simulink model "test_lcl"  (R2021a)
settings: Solver=VariableStepAuto  StartTime=0.0  StopTime=0.2  RelTol=1e-3
values from neighbouring files (symbols this model uses):
  C_a = 1e-3    (= 0.001)    [init.m]
  Lc_a = 0.1    [init.m]
  Lg_a = 1    [init.m]
  Rc_a = 1    [init.m]
  Rf_a = 0.1    [init.m]
  Rg_a = 1    [init.m]
libraries: spsThreePhaseSeriesRLCBranchLib x4, spsThreePhaseVIMeasurementLib x3, spsThreePhaseSourceLib x2, spsMultimeterLib x1, spspowerguiLib x1
settings Model: Creator=viliv  LastModifiedBy=viliv

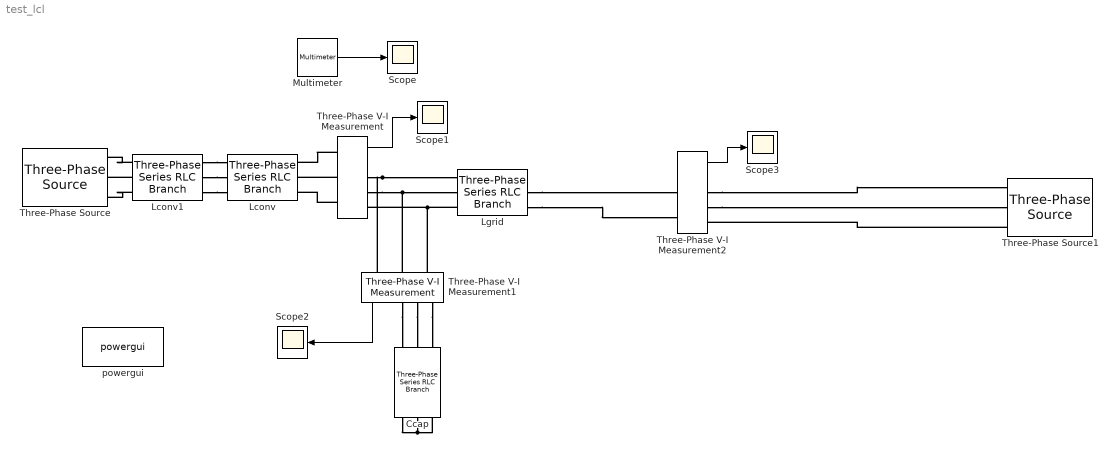
== system test_lcl ==
  Ccap : spsThreePhaseSeriesRLCBranchLib/Three-Phase Series RLC Branch  LConnTagsString=A|B|C  RConnTagsString=A|B|C  BranchType=RC  Resistance=Rf_a  Inductance=2  Capacitance=C_a  Measurements=Branch voltages and currents
  Lconv : spsThreePhaseSeriesRLCBranchLib/Three-Phase Series RLC Branch  LConnTagsString=A|B|C  RConnTagsString=A|B|C  BranchType=L  Resistance=1  Inductance=Lc_a  Capacitance=1e-6  Measurements=Branch voltages and currents
  Lconv1 : spsThreePhaseSeriesRLCBranchLib/Three-Phase Series RLC Branch  LConnTagsString=A|B|C  RConnTagsString=A|B|C  BranchType=R  Resistance=Rc_a  Inductance=0.1  Capacitance=1e-6  Measurements=Branch voltages and currents
  Lgrid : spsThreePhaseSeriesRLCBranchLib/Three-Phase Series RLC Branch  LConnTagsString=A|B|C  RConnTagsString=A|B|C  BranchType=RL  Resistance=Rg_a  Inductance=Lg_a  Capacitance=1e-6  Measurements=Branch voltages and currents
  Multimeter : spsMultimeterLib/Multimeter  PhasorSimulation=off  OutputType=Complex  sel=[4 5 6]  L=24  Gain=[1 1 1]  yselected={'Ub1: Lconv','Ub2: Lconv','Ub3: Lconv'};  PSBOutputType=1  PSBequivalent=0  AxesSetting=[0,0.1,-100,100]  Display=0  SavedBlockNames=-11
  Scope{,1..3} (4 alike) : Scope
  Three-Phase V-I Measurement : spsThreePhaseVIMeasurementLib/Three-Phase V-I Measurement  VoltageMeasurement=phase-to-ground  SetLabelV=off  LabelV=Vabc  Vpu=off  VpuLL=off  CurrentMeasurement=yes  SetLabelI=off  LabelI=Iabc  Ipu=off  Pbase=100e6  Vbase=500e3  OutputType=Complex  PhasorSimulation=off  PSBequivalent=0
  Three-Phase V-I Measurement1 : spsThreePhaseVIMeasurementLib/Three-Phase V-I Measurement  VoltageMeasurement=phase-to-ground  SetLabelV=off  LabelV=Vabc  Vpu=off  VpuLL=off  CurrentMeasurement=yes  SetLabelI=off  LabelI=Iabc  Ipu=off  Pbase=100e6  Vbase=500e3  OutputType=Complex  PhasorSimulation=off  PSBequivalent=0
  Three-Phase V-I Measurement2 : spsThreePhaseVIMeasurementLib/Three-Phase V-I Measurement  VoltageMeasurement=phase-to-ground  SetLabelV=off  LabelV=Vabc  Vpu=off  VpuLL=off  CurrentMeasurement=yes  SetLabelI=off  LabelI=Iabc  Ipu=off  Pbase=100e6  Vbase=500e3  OutputType=Complex  PhasorSimulation=off  PSBequivalent=0
  Three-Phase Source : spsThreePhaseSourceLib/Three-Phase Source  InternalConnection=Y  VoltagePhases=off  Voltage=400 * sqrt(3) / sqrt(2)  PhaseAngle=0  Voltage_phases=[25e3 25e3 25e3]/sqrt(3)  PhaseAngles_phases=[0 -120 +120]  Frequency=50  NonIdealSource=off  SpecifyImpedance=off  Resistance=0.8929  Inductance=16.58e-3  ShortCircuitLevel=100e6  BaseVoltage=25e3  XRratio=7  BusType=swing  Pref=10e3  Qref=0  Prefabc=[10e3, 10e3, 10e3]  Qrefabc=[0, 0, 0]  Qmin=-inf  Qmax=inf
  Three-Phase Source1 : spsThreePhaseSourceLib/Three-Phase Source  InternalConnection=Yg  VoltagePhases=off  Voltage=400 * sqrt(3) / sqrt(2)  PhaseAngle=180  Voltage_phases=[25e3 25e3 25e3]/sqrt(3)  PhaseAngles_phases=[0 -120 +120]  Frequency=50  NonIdealSource=off  SpecifyImpedance=off  Resistance=0.8929  Inductance=16.58e-3  ShortCircuitLevel=100e6  BaseVoltage=25e3  XRratio=7  BusType=swing  Pref=10e3  Qref=0  Prefabc=[10e3, 10e3, 10e3]  Qrefabc=[0, 0, 0]  Qmin=-inf  Qmax=inf
  powergui : spspowerguiLib/powergui  Priority=1  SimulationMode=Discrete  SampleTime=10e-6  frequency=60  Iterations=50  frequencyindice=50  Pbase=100e6  ErrMax=1e-4  UnitsV=kV  UnitsW=MW  buscounter=0  FunctionMessages=off  echomessages=off  EnableUseOfTLC=off  CurrentSourceSwitches=off  DisableSnubberDevices=off  DisableRonSwitches=off  DisableVfSwitches=off  DisplayEquations=off  AutomaticDiscreteSolvers=off  SolverType=Tustin  Interpol=off  ExternalGateDelay=off  methode=off  Ts=100  x0status=zero  SPID=on  SwTol=0  HookPort=off  NonlinearTolerance=1e-6  nMaxIteration=100  ContinueOnMaxIteration=off  RestoreLinks=warning  ResistiveCurrentMeasurement=off  Frange=[0:2:500]  Ylog=off  Xlog=on  ShowGrid=off  save=off  variable=ZData  structure=0  ZoomFFT=off  StartTime=0.0  cycles=1  DisplayStyle=1  fundamental=60  FreqAxis=off  MaxFrequency=1000  frequencyindicesteady=1  RmsSteady=1  display=off
  wires:
  Multimeter/1 -> Scope/1
  Three-Phase V-I Measurement2/1 -> Scope3/1
  Three-Phase V-I Measurement1/1 -> Scope2/1
  Three-Phase V-I Measurement/1 -> Scope1/1
  connections:
  Three-Phase V-I Measurement/RConn2 -- Three-Phase V-I Measurement1/LConn2 -- Lgrid/LConn2
  Ccap/RConn1 -- Ccap/RConn2 -- Ccap/RConn3
  Three-Phase V-I Measurement2/RConn2 -- Three-Phase Source1/RConn2
  Three-Phase V-I Measurement2/RConn1 -- Three-Phase Source1/RConn1
  Three-Phase Source1/RConn3 -- Three-Phase V-I Measurement2/RConn3
  Three-Phase V-I Measurement/LConn2 -- Lconv/RConn2
  Three-Phase V-I Measurement/LConn1 -- Lconv/RConn1
  Three-Phase V-I Measurement/LConn3 -- Lconv/RConn3
  Three-Phase V-I Measurement/RConn1 -- Three-Phase V-I Measurement1/LConn1 -- Lgrid/LConn1
  Lgrid/LConn3 -- Three-Phase V-I Measurement1/LConn3 -- Three-Phase V-I Measurement/RConn3
  Three-Phase V-I Measurement1/RConn1 -- Ccap/LConn1
  Three-Phase V-I Measurement1/RConn2 -- Ccap/LConn2
  Three-Phase V-I Measurement1/RConn3 -- Ccap/LConn3
  Lconv1/LConn2 -- Three-Phase Source/RConn2
  Lconv1/RConn1 -- Lconv/LConn1
  Lconv1/RConn2 -- Lconv/LConn2
  Lconv1/RConn3 -- Lconv/LConn3
  Lconv1/LConn1 -- Three-Phase Source/RConn1
  Lconv1/LConn3 -- Three-Phase Source/RConn3
  Lgrid/RConn3 -- Three-Phase V-I Measurement2/LConn3
  Lgrid/RConn2 -- Three-Phase V-I Measurement2/LConn2
